simulink model "Nolimitation_Model"  (R2018a)
settings: Solver=VariableStepAuto  StartTime=0.0  StopTime=10.0  RelTol=1e-3
values from neighbouring files (symbols this model uses):
  KT = 0.25    [DC_Motormfile.m]    (also in pid.m)
  L = 493*10^-9    (= 4.93e-07)    [DC_Motormfile.m]    (also in pid.m)
  R = 5.3*10^-3    (= 0.0053)    [DC_Motormfile.m]    (also in pid.m)
  Scaling_Velocity = Sc/(Cw)*Rg*KE    (= 4.865)    [pid.m]
  Ts = 0.01    [pid.m]
settings Model: Creator=MAFAZ  LastModifiedBy=MAFAZ

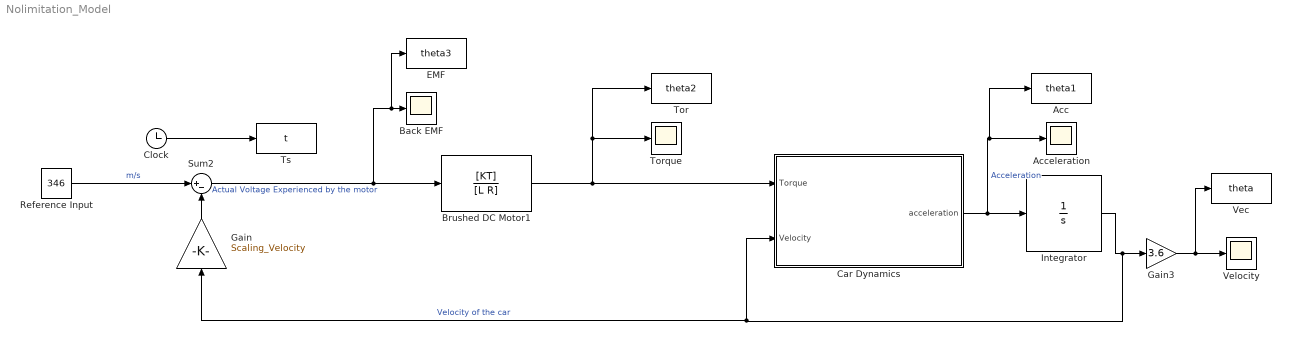
== system Nolimitation_Model ==
  Acc : ToWorkspace  VariableName=theta1  SampleTime=Ts
  Acceleration : Scope
  Back EMF : Scope
  Brushed DC Motor1 : TransferFcn  Numerator=[KT]  Denominator=[L R]
  Car Dynamics : MATLAB Function  TreatAsAtomicUnit=on
  Clock : Clock
  EMF : ToWorkspace  VariableName=theta3  SampleTime=Ts
  Gain : Gain  Gain=Scaling_Velocity
  Gain3 : Gain  Gain=3.6
  Integrator : Integrator
  Reference Input : Constant  Value=346
  Sum2 : Sum  Inputs=|+-
  Tor : ToWorkspace  VariableName=theta2  SampleTime=Ts
  "Torque " : Scope
  Ts : ToWorkspace  VariableName=t  SampleTime=Ts
  Vec : ToWorkspace  VariableName=theta  SampleTime=Ts
  Velocity : Scope
  wires:
  Sum2/1 -> Brushed DC Motor1/1, EMF/1, Back EMF/1  "Actual Voltage Experienced by the motor"
  Gain3/1 -> Vec/1, Velocity/1
  Reference Input/1 -> Sum2/1  "m/s"
  Car Dynamics/1(acceleration) -> Acc/1, Acceleration/1, Integrator/1  "Acceleration"
  Integrator/1 -> Gain/1, Car Dynamics/2(Velocity), Gain3/1  "Velocity of the car"
  Gain/1 -> Sum2/2
  Clock/1 -> Ts/1
  Brushed DC Motor1/1 -> Car Dynamics/1(Torque), Tor/1, "Torque "/1

== matlab function Nolimitation_Model/Car Dynamics ==
  data: Torque input; acceleration output; Velocity input
function acceleration = fcn(Torque, Velocity)
acceleration = (40.5*Torque*0.6-413-0.3381*Velocity^2)/2108;

% 0.6 = mechanical efficiency of the vehcile - to ensure its reaches 100
% km/h within 4.4 secs. 

% 413 = actual Rolling Resistance 
%0.3381 = drag force created by the movement of the car

%2108 = mass of the car
